simulink model "A_Canary"  (Simulink 8.1)
settings: Solver=ode4  StartTime=0.0  StopTime=inf  FixedStep=Ts  MaxStep=1e-3  RelTol=1e-3
PostLoadFcn:
  | Canary_init;
InitFcn:
  | Canary_init;
values from neighbouring files (symbols this model uses):
  f = 60    [Software_BESS_init.m]
  filt = firstOrderDig(50e-3, Tc, 'low')    [Software_BESS_init.m]    (also in firstOrderDig.m = (tau*s) / (tau*s + 1))
  Igrid = Pgrid/Vgrid/3    [Software_BESS_init.m]
  paramDroopFreq2Reac = 0.5*(1/0.05)    (= 10)    [Software_BESS_init.m]
  paramDroopFreq2Real = 0*(1/0.05)    (= 0)    [Software_BESS_init.m]
  paramDroopVolts2Reac = 0*(1/0.05)    (= 0)    [Software_BESS_init.m]
  paramDroopVolts2Real = 0.5*(1/0.05)    (= 10)    [Software_BESS_init.m]
  paramPLLControlD = 1    [Software_BESS_init.m]
  paramPLLControlI = 320    [Software_BESS_init.m]
  paramPLLControlP = 18    [Software_BESS_init.m]
  Tc = Ts    (= 0.0001)    [Software_BESS_init.m]
  Ts = 100e-6    (= 0.0001)    [Software_BESS_init.m]
  Vgrid = 480/sqrt(3)    [Software_BESS_init.m]
undefined symbols (not defined in the file or in its folder): cable_spec, fdesignblkfcn, gcbh, generic_ethernet_cb, HWController_3, HWController_NG_Generator, HWController_NG_Genset_3, HWController_NGCHP_Genset_3p5MVA_lib, Left, relay_par, SEL751, SEL751_SignalScaling_lib, SignalScaling, type, V
libraries: powerlib_extras x16, powerlib x15, rtlab x10, rtio_opalrt_common x10, cables_lib x6, rtio_opalrt_op5142ex1 x6, powerlib_meascontrol x5, simulink x5, breaker_lib x4, simulink_extras x4, rtio_generic_modbus x3, ssn_lib x2
(part 4 of 4)

== system A_Canary/SM_system/HWController_3.5MVA_NGCHP/HWController_NG_Generator/HWController_NG_Genset_3.5MVA/3.5MVA Generator with  Primary Controllers/NG Engine Speed & Voltage Control fast/Excitation1/Damping kf.s / (tf.s +1)/1st-Order Discrete Filter ==
  In : Inport
  Discrete State-Space : DiscreteStateSpace  A=Ad  B=Bd  C=Cd  D=Dd  X0=x0d  SampleTime=Ts
  Out : Outport  InitialOutput=0
  wires:
  In/1 -> Discrete State-Space/1
  Discrete State-Space/1 -> Out/1

== system A_Canary/SM_system/HWController_3.5MVA_NGCHP/HWController_NG_Generator/HWController_NG_Genset_3.5MVA/3.5MVA Generator with  Primary Controllers/NG Engine Speed & Voltage Control fast/Excitation1/Exciter  1 / (te.s + ke)/1st order Lowpass ==
  In : Inport
  Discrete State-Space : DiscreteStateSpace  A=Ad  B=Bd  C=Cd  D=Dd  X0=x0d  SampleTime=Ts
  Out : Outport  InitialOutput=0
  wires:
  In/1 -> Discrete State-Space/1
  Discrete State-Space/1 -> Out/1

== system A_Canary/SM_system/HWController_3.5MVA_NGCHP/HWController_NG_Generator/HWController_NG_Genset_3.5MVA/3.5MVA Generator with  Primary Controllers/NG Engine Speed & Voltage Control fast/Excitation1/Main Regulator ka / (ta.s +1)/1st order Lowpass ==
  In : Inport
  Discrete State-Space : DiscreteStateSpace  A=Ad  B=Bd  C=Cd  D=Dd  X0=x0d  SampleTime=Ts
  Out : Outport  InitialOutput=0
  wires:
  In/1 -> Discrete State-Space/1
  Discrete State-Space/1 -> Out/1
